simulink model "power_quality_analyzer"  (R2025b)
settings: Solver=VariableStepAuto  StartTime=0.0  StopTime=3  RelTol=1e-3
libraries: simulink x6, dspstat3 x3, hdlsllib x1
settings Model: Creator=urshi  LastModifiedBy=urshi

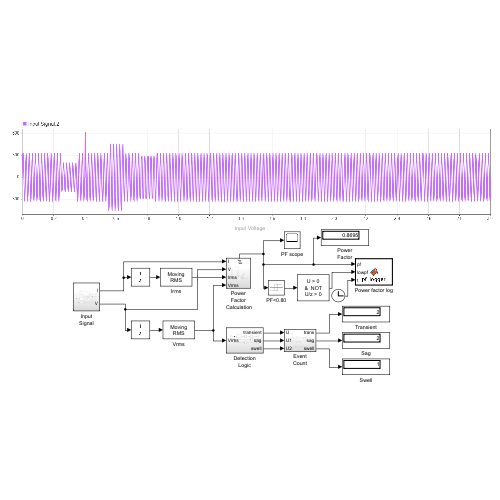
[thumbnail: Simulink's stored preview of the top-level diagram]
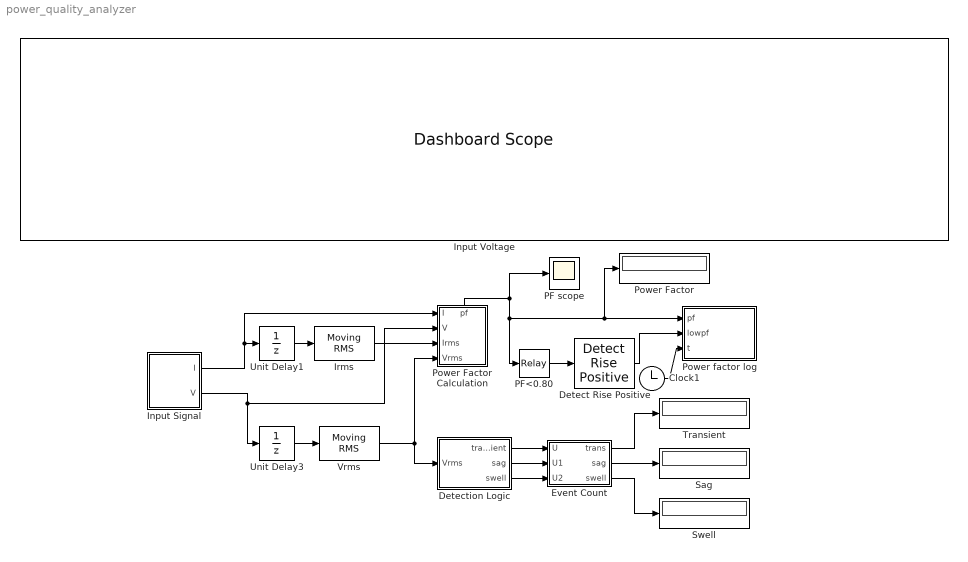
== system power_quality_analyzer ==
  Clock1 : Clock
  Detect Rise Positive : simulink/Logic and Bit Operations/Detect Rise Positive  vinit=0  OutDataTypeStr=boolean
  Detection Logic : Subsystem
  Event Count : Subsystem
  Input Signal : Subsystem
  Input Voltage : DashboardScope  FontColor=[0.0, 0.0, 0.0]
  Irms : dspstat3/Moving RMS  Method=Sliding window  ForgettingFactorPort=off  SpecifyWindowLength=on  WindowLength=200  OverlapLength=199  AllowArbitraryInputLength=off  ForgettingFactor=0.9  SimulateUsing=Interpreted execution
  PF scope : Scope
      settings: ActiveDisplayYMinimum=0.49142671409023336  ActiveDisplayYMaximum=1.1711119795565292  DataLoggingVariableName=ScopeData4
  PF<0.80 : Relay  OnSwitchValue=0.85  OffSwitchValue=0.80  OnOutputValue=0  OffOutputValue=1
  Power Factor : Display
  Power Factor Calculation : Subsystem
      settings: PortSchema="{\"entries\":[{\"content\":{\"sides\":[{\"content\":{\"connectorIds\":[\"In1\",\"In2\",\"In3\",\"In4\"]},\"type\":\"ConnectorPlacement.EquallySpacedRectSide\",\"uuid\":\"a45e54df-5af6-4526-ba1e-c0a636d7952d\"},{\"content\":{\"side\":\"RIGHT\"},\"type\":\"ConnectorPlacement.EquallySpacedRectSide\",\"uuid\":\"751388e3-94d5-4227-ac80-4fdd0b43f594\"},{\"content\":{\"connectorIds\":[\"Out1\"],\"side\":\"TOP\"},\"type\":\"ConnectorPlacement.EquallySpacedRectSide\",\"uuid\":\"7513935c-f989-4ca5-8507-f010a8684484\"}]},\"type\":\"ConnectorPlacement.EquallySpacedConnector\",\"uuid\":\"c5c7e349-e438-4b16-8b4f-27dae6d22da7\"}],\"packageUris\":[\"http://schema.mathworks.com/mf0/Connector/R2020b\"],\"version\":\"1.0\"}"
  Power factor log : MATLAB Function  TreatAsAtomicUnit=on
  Sag : Display
  Swell : Display
  Transient : Display
  Unit Delay1 : UnitDelay  SampleTime=-1  HasFrameUpgradeWarning=on
  Unit Delay3 : UnitDelay  SampleTime=-1  HasFrameUpgradeWarning=on
  Vrms : dspstat3/Moving RMS  Method=Sliding window  ForgettingFactorPort=off  SpecifyWindowLength=on  WindowLength=200  OverlapLength=199  AllowArbitraryInputLength=off  ForgettingFactor=0.9  SimulateUsing=Interpreted execution
  wires:
  Input Signal/2(V) -> Unit Delay3/1, Power Factor Calculation/2(V)
  Unit Delay3/1 -> Vrms/1
  Vrms/1 -> Detection Logic/1(Vrms), Power Factor Calculation/4(Vrms)
  Event Count/1(trans) -> Transient/1
  Event Count/2(sag) -> Sag/1
  Event Count/3(swell) -> Swell/1
  Input Signal/1(I) -> Power Factor Calculation/1(I), Unit Delay1/1
  PF<0.80/1 -> Detect Rise Positive/1
  Detect Rise Positive/1 -> Power factor log/2(lowpf)
  Power Factor Calculation/1(pf) -> PF<0.80/1, Power Factor/1, Power factor log/1(pf), PF scope/1
  Irms/1 -> Power Factor Calculation/3(Irms)
  Unit Delay1/1 -> Irms/1
  Clock1/1 -> Power factor log/3(t)
  Detection Logic/1(transient) -> Event Count/1(U)
  Detection Logic/2(sag) -> Event Count/2(U1)
  Detection Logic/3(swell) -> Event Count/3(U2)

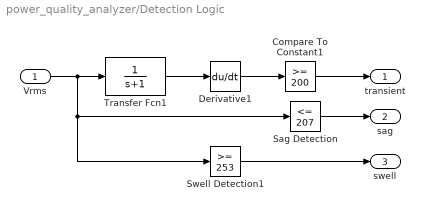
== system power_quality_analyzer/Detection Logic ==
  Vrms : Inport
  Compare To Constant1 : simulink/Logic and Bit Operations/Compare To Constant  relop=>=  const=200  OutDataTypeStr=boolean
  Derivative1 : Derivative
  Sag Detection : simulink/Logic and Bit Operations/Compare To Constant  relop=<=  const=207  OutDataTypeStr=boolean
  Swell Detection1 : simulink/Logic and Bit Operations/Compare To Constant  relop=>=  const=253  OutDataTypeStr=boolean
  Transfer Fcn1 : TransferFcn  Denominator=[1 1]
  transient : Outport
  sag : Outport  Port=2
  swell : Outport  Port=3
  wires:
  Transfer Fcn1/1 -> Derivative1/1
  Vrms/1 -> Swell Detection1/1, Sag Detection/1, Transfer Fcn1/1
  Derivative1/1 -> Compare To Constant1/1
  Sag Detection/1 -> sag/1
  Compare To Constant1/1 -> transient/1
  Swell Detection1/1 -> swell/1

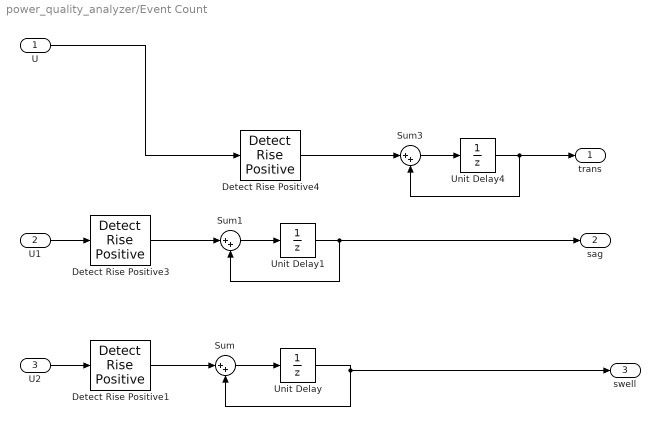
== system power_quality_analyzer/Event Count ==
  U : Inport
  U1 : Inport  Port=2
  U2 : Inport  Port=3
  Detect Rise Positive1 : simulink/Logic and Bit Operations/Detect Rise Positive  vinit=0  OutDataTypeStr=uint8
  Detect Rise Positive3 : hdlsllib/Logic and Bit Operations/Detect Rise Positive  vinit=0  OutDataTypeStr=uint8
  Detect Rise Positive4 : simulink/Logic and Bit Operations/Detect Rise Positive  vinit=0  OutDataTypeStr=uint8
  Sum : Sum  Inputs=|++
  Sum1 : Sum  Inputs=|++
  Sum3 : Sum  Inputs=|++
  Unit Delay : UnitDelay  SampleTime=-1  HasFrameUpgradeWarning=on
  Unit Delay1 : UnitDelay  SampleTime=-1  HasFrameUpgradeWarning=on
  Unit Delay4 : UnitDelay  SampleTime=-1  HasFrameUpgradeWarning=on
  trans : Outport
  sag : Outport  Port=2
  swell : Outport  Port=3
  wires:
  U/1 -> Detect Rise Positive4/1
  Sum1/1 -> Unit Delay1/1
  Detect Rise Positive3/1 -> Sum1/1
  Unit Delay/1 -> swell/1, Sum/2
  Detect Rise Positive1/1 -> Sum/1
  Sum/1 -> Unit Delay/1
  Detect Rise Positive4/1 -> Sum3/1
  Unit Delay1/1 -> sag/1, Sum1/2
  Unit Delay4/1 -> trans/1, Sum3/2
  Sum3/1 -> Unit Delay4/1
  U2/1 -> Detect Rise Positive1/1
  U1/1 -> Detect Rise Positive3/1

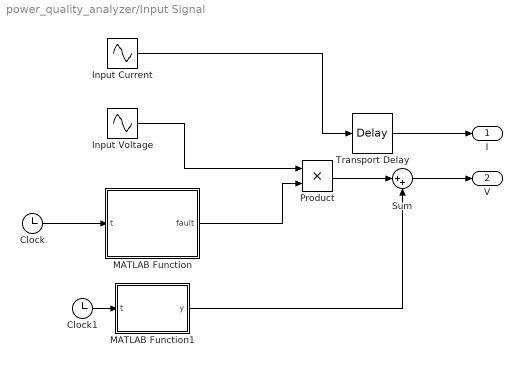
== system power_quality_analyzer/Input Signal ==
  Clock : Clock
  Clock1 : Clock
  Input Current : Sin  Amplitude=8  Frequency=2*50*pi  SampleTime=0.0002
  Input Voltage : Sin  Amplitude=325.27  Frequency=2*50*pi  SampleTime=0.0002
  MATLAB Function : MATLAB Function  TreatAsAtomicUnit=on
  MATLAB Function1 : MATLAB Function  TreatAsAtomicUnit=on
  Product : Product
  Sum : Sum  Inputs=|++
  Transport Delay : TransportDelay  DelayTime=0.00167
  I : Outport
  V : Outport  Port=2
  wires:
  Input Voltage/1 -> Product/1
  Clock/1 -> MATLAB Function/1(t)
  MATLAB Function/1(fault) -> Product/2
  Product/1 -> Sum/1
  Sum/1 -> V/1
  Clock1/1 -> MATLAB Function1/1(t)
  MATLAB Function1/1(y) -> Sum/2
  Input Current/1 -> Transport Delay/1
  Transport Delay/1 -> I/1

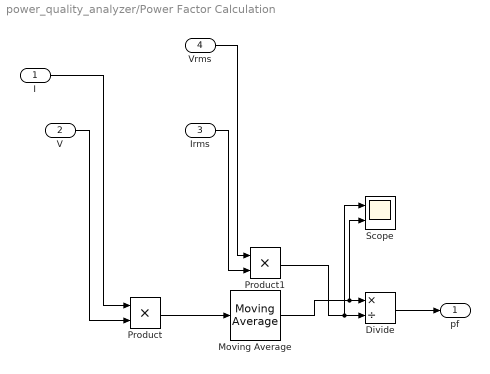
== system power_quality_analyzer/Power Factor Calculation ==
  I : Inport
  V : Inport  Port=2
  Irms : Inport  Port=3
  Vrms : Inport  Port=4
  Divide : Product  Inputs=*/
  Moving Average : dspstat3/Moving Average  Method=Sliding window  ForgettingFactorPort=off  SpecifyWindowLength=off  WindowLength=200  OverlapLength=199  AllowArbitraryInputLength=off  ForgettingFactor=0.9  SimulateUsing=Interpreted execution
  Product : Product
  Product1 : Product
  Scope : Scope  NumInputPorts=2
      settings: ActiveDisplayYMinimum=-362.57733374671079  ActiveDisplayYMaximum=3049.0749343517737
  pf : Outport
  wires:
  Divide/1 -> pf/1
  Vrms/1 -> Product1/1
  Irms/1 -> Product1/2
  Product1/1 -> Scope/1, Divide/2
  I/1 -> Product/1
  V/1 -> Product/2
  Product/1 -> Moving Average/1
  Moving Average/1 -> Scope/2, Divide/1

== matlab function power_quality_analyzer/Power factor log ==
  data: pf input; lowpf input; t input
function pf_logger(pf, lowpf, t)

persistent prev_lowpf

if isempty(prev_lowpf)
    prev_lowpf = 0;
end

if t > 0.05 && lowpf && ~prev_lowpf
    fprintf('LOW PF: %.2f at %.2f s\n', pf, t);
end

== matlab function power_quality_analyzer/Input Signal/MATLAB Function ==
  data: t input; fault output
function fault = fault_injector(t)

fault = 1;   % normal voltage (no fault)

if t > 0.25 && t < 0.35
    fault = 0.6;     % voltage sag
end

if t > 0.55 && t < 0.65
    fault = 1.4;     % voltage swell

end

== matlab function power_quality_analyzer/Input Signal/MATLAB Function1 ==
  data: t input; y output
function y = fcn(t)

y = 1;

% TRANSIENT (short spike)
if t >= 0.40 && t <= 0.405
    y= 300*sin(2*pi*2000*t);
end

% HARMONIC (3rd harmonic distortion)
if t >= 0.75 && t <= 0.85
    y= 0.2*325*sin(2*pi*3*50*t);
end
